simulink model "Trajektorien_test"  (R2020a)
settings: Solver=FixedStepAuto  StartTime=0.0  StopTime=10.0  FixedStep=0.01  RelTol=1e-3
settings Model: Creator=Frederik  LastModifiedBy=Tobias

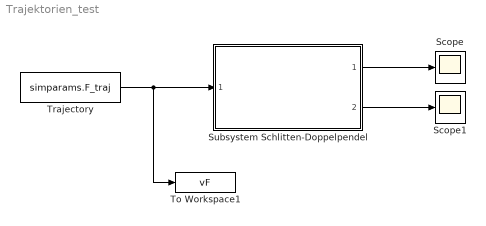
== system Trajektorien_test ==
  Scope : Scope
  Scope1 : Scope
  Subsystem Schlitten-Doppelpendel : Subsystem  ReferencedSubsystem=SchlittenPendel  params=simparams.gesamtmodell.schlittenpendel
  To Workspace1 : ToWorkspace  VariableName=vF  SaveFormat=Timeseries  SampleTime=-1
  Trajectory : FromWorkspace  VariableName=simparams.F_traj  Interpolate=off  OutputAfterFinalValue=Setting to zero
  wires:
  Subsystem Schlitten-Doppelpendel/2 -> Scope1/1
  Trajectory/1 -> To Workspace1/1, Subsystem Schlitten-Doppelpendel/1
  Subsystem Schlitten-Doppelpendel/1 -> Scope/1
